simulink model "WhiteNoiseTorque"  (R2024b)
settings: Solver=FixedStepAuto  StartTime=0.0  StopTime=10.0  RelTol=1e-3
undefined symbols (not defined in the file or in its folder): simu
libraries: simulink x1
settings Model: Creator=jackson  LastModifiedBy=jackson

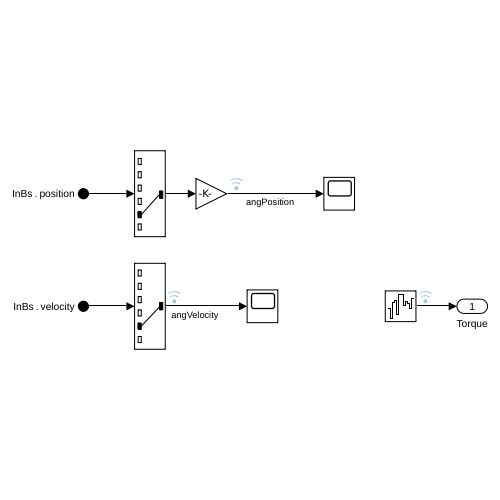
[thumbnail: Simulink's stored preview of the top-level diagram]
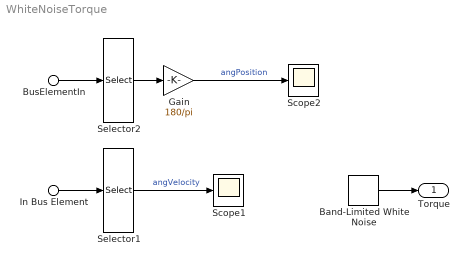
== system WhiteNoiseTorque ==
  In Bus Element : Inport  PortName=InBs  Element=velocity
  BusElementIn : Inport  PortName=InBs  Element=position
  Band-Limited White Noise : simulink/Sources/Band-Limited White Noise  Cov=1e6  Ts=simu.dt  seed=[23341]
  Gain : Gain  Gain=180/pi
  Scope1 : Scope
  Scope2 : Scope
  Selector1 : Selector  InputPortWidth=6  IndexOptions=Index vector (dialog)  Indices=5  OutputSizes=1
  Selector2 : Selector  InputPortWidth=6  IndexOptions=Index vector (dialog)  Indices=5  OutputSizes=1
  Torque : Outport
  wires:
  Band-Limited White Noise/1 -> Torque/1
  Selector1/1 -> Scope1/1  "angVelocity"
  In Bus Element/1 -> Selector1/1
  BusElementIn/1 -> Selector2/1
  Selector2/1 -> Gain/1
  Gain/1 -> Scope2/1  "angPosition"
